simulink model "check"  (R2023b)
settings: Solver=VariableStepAuto  StartTime=0.0  StopTime=inf  RelTol=1e-3
libraries: fuzblock x1
settings Model: Creator=trucd  LastModifiedBy=trucd

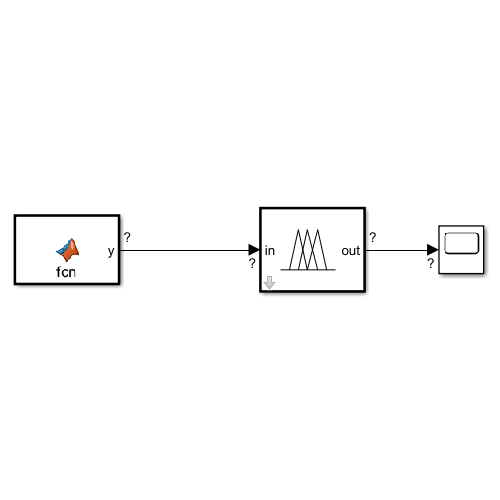
[thumbnail: Simulink's stored preview of the top-level diagram]
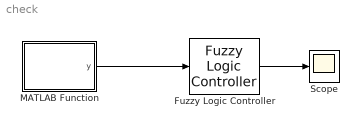
== system check ==
  Fuzzy Logic Controller : fuzblock/Fuzzy Logic  Controller  FIS='Fuzzy_Model.fis'  OutputSampleNumber=101  DataType=double  FuzzifiedInputs=off  RuleFiringStrengths=off  RuleOutputs=off  AggregatedOutputs=off  SimulateUsing=Interpreted execution  OutOfRangeInputValueMessage=warning  NoRuleFiredMessage=warning  EmptyOutputFuzzySetMessage=warning
  MATLAB Function : MATLAB Function  TreatAsAtomicUnit=on
  Scope : Scope
  wires:
  Fuzzy Logic Controller/1 -> Scope/1
  MATLAB Function/1(y) -> Fuzzy Logic Controller/1

== matlab function check/MATLAB Function ==
  data: y output
function y = fcn()
data = thingSpeakRead(2327722,'Fields',1,NumPoints=1);
y = data;
